simulink model "husky_sim - Copy"  (R2019b)
settings: Solver=ode4  StartTime=0.0  StopTime=3  FixedStep=0.006  RelTol=1e-3
InitFcn:
  | init_model;
values from neighbouring files (symbols this model uses):
  m = getfield(leg,'mass')    [dynamic_test.m]    (also in pen_init.m = link2.mass; test.mat = 2.2337)
  q_BL_K0 = initial_angle(12)    [func_params_ext.m]
  q_BR_K0 = initial_angle(9)    [func_params_ext.m]
  q_FL_K0 = initial_angle(6)    [func_params_ext.m]
undefined symbols (not defined in the file or in its folder): body, femur_left, femur_right, hip_left, hip_right, link_left, link_right, tarsus_left, tarsus_right, tibia_left, tibia_right, X, Y, Z
libraries: sm_lib x206, nesl_utility x56, dspsigops x7, Contact_Forces_Lib x4, simulink x2
(part 6 of 6)

== matlab function husky_sim - Copy/Foot placement/husky_FK ==
  data: q_curr input; p_end_req output double size=[12,1]; leg_params parameter
% Find current leg end position based on encoder readings (in reads)
%
% Inputs: 
%   q_curr - (12x1) current joint angles in the following order
%       [q_FR_HF; q_FR_HS; q_FR_K;
%       q_FL_HF; q_FL_HS; q_FL_K
%       q_BR_HF; q_BR_HS; q_BR_K
%       q_BL_HF; q_BL_HS; q_BL_K]
% 
% Prameters: 
%   leg_params - parameters needed for computing FK or IK in each leg
%       [l_hip_offset, l1, l2, l3, q_hf_offset, q_hs_offset, q_k_offset]
%       (see notes)
%   backbone_mass_pos_wrt_body - location [x,y,z] of backbone mass 
%       relative to body cooridnate frame
%   body - structure which contains mass and inertial properties of backbone
%           used to obtain body mass
%   hip_orgin_wrt_backbone - (1x12) position [x,y,z] of hip coordinate frame of
%       each leg relative to body
%   femur_left - structure which contains mass and inertial properties of
%       femur used to obtain mass of femur (same for lef and right femur)
%   femur_mass_loc - (12x1) location [x,y,z] of all 4 femur mass relative to 
%   	hip reference frame
%
% Output: 
%   p_end_req - (12x1) feet end positions [FR, FL, BR, BL] relative to 
%           respsective leg hip coordinate frame
%
% NOTES: 
%
% By Pravin Dangol, 12-05-19 (approx), Boston, MA
function p_end_req = func_husky_FK(q_curr, leg_params)

q_curr_FR = q_curr(1:3);
q_curr_FL = q_curr(4:6);
q_curr_BR = q_curr(7:9);
q_curr_BL = q_curr(10:12);

p_end_FR_curr = func_FK_right(q_curr_FR,leg_params);
p_end_FL_curr = func_FK_left(q_curr_FL,leg_params);
p_end_BR_curr = func_FK_right(q_curr_BR,leg_params);
p_end_BL_curr = func_FK_left(q_curr_BL,leg_params);

p_end_req = [p_end_FR_curr; p_end_FL_curr; p_end_BR_curr; p_end_BL_curr];

end

function p_end = func_FK_right(q,leg_param)
%FUNC_FK
%    P_END = FUNC_FK(IN1,IN2)

%    This function was generated by the Symbolic Math Toolbox version 8.3.
%    12-Dec-2019 10:24:24

% Right leg FK
% Obtain feet end position [x, y, z] based on leg angles [q_hf, q_hs, q_k]
%
% Inputs: q = [q_hf, q_hs, q_k]; hip frontal, hip sagittal and knee angles
%         leg_params = [l_offset l1 l2 l3] leg lengths (see notes)
%
% Output: p_end = [x; y; z] coordinates of feet end
% by Pravin Dangol, Boston, MA
l1 = leg_param(2);
l2 = leg_param(3);
l3 = leg_param(4);
l_offset = leg_param(1);
q_hf = q(1);
q_hs = q(2);
q_k = q(3);
q_hf_offset = leg_param(5);
q_hs_offset = leg_param(6);
q_k_offset = leg_param(7);
p_end = [-l2.*sin(q_hs+q_k+q_hs_offset+q_k_offset)+l1.*sin(q_hs+q_hs_offset)+l3.*sin(q_hs+q_hs_offset);...
    l_offset.*sin(q_hf-q_hf_offset)-l1.*cos(q_hf-q_hf_offset).*cos(q_hs+q_hs_offset)-l3.*cos(q_hf-q_hf_offset).*cos(q_hs+q_hs_offset)+l2.*cos(q_hf-q_hf_offset).*cos(q_hs+q_hs_offset).*cos(q_k+q_k_offset)-l2.*cos(q_hf-q_hf_offset).*sin(q_hs+q_hs_offset).*sin(q_k+q_k_offset);...
    l_offset.*cos(q_hf-q_hf_offset)+l1.*sin(q_hf-q_hf_offset).*cos(q_hs+q_hs_offset)+l3.*sin(q_hf-q_hf_offset).*cos(q_hs+q_hs_offset)-l2.*sin(q_hf-q_hf_offset).*cos(q_hs+q_hs_offset).*cos(q_k+q_k_offset)+l2.*sin(q_hf-q_hf_offset).*sin(q_hs+q_hs_offset).*sin(q_k+q_k_offset)];

% p_end = reshape(p_end,1,12);

end

function p_end = func_FK_left(q,leg_param)
%FUNC_FK_LEFT
%    P_END = FUNC_FK_LEFT(IN1,IN2)

%    This function was generated by the Symbolic Math Toolbox version 8.3.
%    12-Dec-2019 10:24:24

% Left leg FK
% Obtain feet end position [x, y, z] based on leg angles [q_hf, q_hs, q_k]
%
% Inputs: q = [q_hf, q_hs, q_k]; hip frontal, hip sagittal and knee angles
%         leg_params = [l_offset l1 l2 l3] leg lengths (see notes)
%
% Output: p_end = [x; y; z] coordinates of feet end
% by Pravin Dangol, Boston, MA
l1 = leg_param(2);
l2 = leg_param(3);
l3 = leg_param(4);
l_offset = leg_param(1);
q_hf = q(1);
q_hs = q(2);
q_k = q(3);
q_hf_offset = leg_param(5);
q_hs_offset = leg_param(6);
q_k_offset = leg_param(7);
p_end = [-l2.*sin(q_hs+q_k+q_hs_offset+q_k_offset)+l1.*sin(q_hs+q_hs_offset)+l3.*sin(q_hs+q_hs_offset);...
    -l_offset.*sin(q_hf-q_hf_offset)+l1.*cos(q_hf-q_hf_offset).*cos(q_hs+q_hs_offset)+l3.*cos(q_hf-q_hf_offset).*cos(q_hs+q_hs_offset)-l2.*cos(q_hf-q_hf_offset).*cos(q_hs+q_hs_offset).*cos(q_k+q_k_offset)+l2.*cos(q_hf-q_hf_offset).*sin(q_hs+q_hs_offset).*sin(q_k+q_k_offset);...
    l_offset.*cos(q_hf-q_hf_offset)+l1.*sin(q_hf-q_hf_offset).*cos(q_hs+q_hs_offset)+l3.*sin(q_hf-q_hf_offset).*cos(q_hs+q_hs_offset)-l2.*sin(q_hf-q_hf_offset).*cos(q_hs+q_hs_offset).*cos(q_k+q_k_offset)+l2.*sin(q_hf-q_hf_offset).*sin(q_hs+q_hs_offset).*sin(q_k+q_k_offset)];

end

== matlab function husky_sim - Copy/Foot placement/Gait timing/Dynamic gait ==
  data: t input; t_start input; y output; T_f input; Ts parameter
% Generate symmetric triangle waves, with amplitude fixed at 1
%
% Input: t_in = clock time;
%       T_f = desired time to peak
%
% Output: triangle wave
function y = func_triangle_wave(t, t_start, T_f, Ts)

% The general triangle wave formula is used:  
%   y = -2*A/p*abs(mod(t,p)-p/2) + A;
%

time = t - t_start;

% Period
p = T_f*2;
% Amplitude, the same as T_f, so the slope is 1
A = T_f;

y = -2*A/p*abs(mod(time,p)-p/2) + A - Ts;

end

== matlab function husky_sim - Copy/Foot placement/Gait timing/Transition gait ==
  data: t input; y output; t_start input; T_f input; Ts parameter
% Ramp with upper timit, used to create a timing for a trajectory that
% moves from point A to B only once and stops at point B
%
% Inputs: t - clock time,
%       t_start -  time at which start command is given (from sample and
%           hold)
%       T_f - length of time for trajectory 
%       T_s (param) sample time of system
%
% Output: y = x (ramp starting at 0) with slope of 1 until T_f is reached, 
%        then it saturates at T_f
%       This is because the cubic trajectory os only defined from 0 to T_f
%
function y = func_saturated_ramp(t,t_start,T_f, Ts)

% subtracting Ts because the delay in sample and hold adds 1 Ts to time,
% the multiplier of 0.01 ensure zero crossover to activate rising trigger
time = t - t_start - Ts*1.01;

if time < T_f
    y = time;
else 
    y = T_f;
end
    
end

== matlab function husky_sim - Copy/Foot placement/Gait timing/check_transition_end_reached ==
  data: reset_start_time input; y output; switch_to_dynamic input; T_f input; gait_timing input
% Check if end of transition trajectory reached, then reset p0 to current
% reading based off of FK, does not reset for dynamic
%   This ensures, there is no jump in position as start (p0) and end (pf)
%   of trajecotry are the same.
%
% Inputs: reset_start_time: 0 to reset, 1 to start chosen trajectory
%       switch_dynamic: 0 for trasition gait (one shot p0 to pf trajectory)
%                       1 for dynamic (back and forth between two points)
%       T_f: Time taken to reach end of trajecotry
%       gait_timing: timing of chosen trajectory
%
%   Output: 0 of gait not reached, 1 if reached, this activates a rising
%   sample and hold trigger
%
function y = fcn(reset_start_time, switch_to_dynamic, T_f, gait_timing)

if reset_start_time >=1 && switch_to_dynamic == 0 && gait_timing >= T_f 
    y = 1;
else
    y = 0;
end

end
